simulink model "Multiphase_Buck"  (Simulink 6.1)
settings: Solver=ode23tb  SolverMode=SingleTasking  StartTime=0.0  StopTime=0.03  MaxStep=10e-6  RelTol=1e-3
libraries: powerlib x14
settings Model: Creator=patrice  LastModifiedBy=ThinkPad  ExtModeTrigMode=oneshot  ExtModeArmWhenConnect=off  ExtModeAutoUpdateStatusClock=off
settings DataIOCC: LimitDataPoints=off  SignalLoggingName=sigsOut
settings OptimizationCC: BooleanDataType=off
settings HardwareCC: TargetUnknown=on
settings RTWCC: TemplateMakefile=grt_unix.tmf

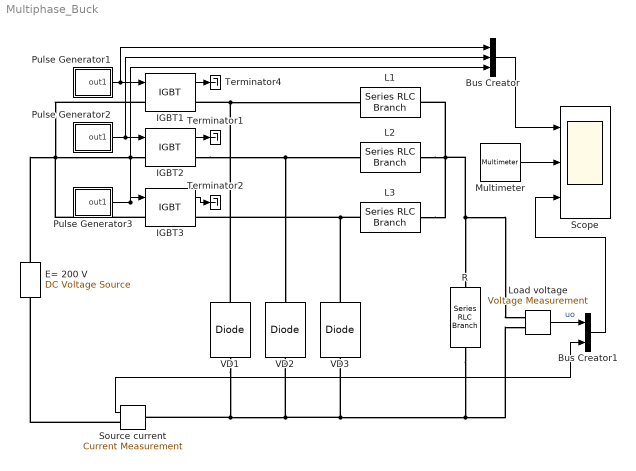
== system Multiphase_Buck ==
  Bus Creator : BusCreator  DialogController=Simulink.DDGSource_Bus  Inputs=3
  Bus Creator1 : BusCreator  DialogController=Simulink.DDGSource_Bus  Inputs=2
  E= 200 V : powerlib/Electrical Sources/DC Voltage Source  Description=source block  Orientation=up  Amplitude=200  Measurements=None
      settings: AttributesFormatString=\n
  IGBT1 : powerlib/Power Electronics/IGBT  Ron=0.5  Lon=1e-6  Vf=0  Tf=1e-6  Tt=1e-6  IC=0  Rs=10  Cs=1e-7  Measurements=on
      settings: AttributesFormatString=\n
  IGBT2 : powerlib/Power Electronics/IGBT  Ron=0.5  Lon=1e-6  Vf=0  Tf=1e-6  Tt=1e-6  IC=0  Rs=10  Cs=1e-7  Measurements=on
      settings: AttributesFormatString=\n
  IGBT3 : powerlib/Power Electronics/IGBT  Ron=0.5  Lon=1e-6  Vf=0  Tf=1e-6  Tt=1e-6  IC=0  Rs=10  Cs=1e-7  Measurements=on
      settings: AttributesFormatString=\n
  L1 : powerlib/Elements/Series RLC Branch  PhysicalDomain=powersysdomain  SubClassName=unknown  LeftPortType=p1  RightPortType=p1  LConnTagsString=__new0  RConnTagsString=__new0  Resistance=0  Inductance=5e-03  Capacitance=inf  Measurements=Branch current
  L2 : powerlib/Elements/Series RLC Branch  PhysicalDomain=powersysdomain  SubClassName=unknown  LeftPortType=p1  RightPortType=p1  LConnTagsString=__new0  RConnTagsString=__new0  Resistance=0  Inductance=5e-03  Capacitance=inf  Measurements=Branch current
  L3 : powerlib/Elements/Series RLC Branch  PhysicalDomain=powersysdomain  SubClassName=unknown  LeftPortType=p1  RightPortType=p1  LConnTagsString=__new0  RConnTagsString=__new0  Resistance=0  Inductance=5e-03  Capacitance=inf  Measurements=Branch current
  Load voltage : powerlib/Measurements/Voltage Measurement  Tag=PoWeRsYsTeMmEaSuReMeNt  PhasorSimulation=off  OutputType=Magnitude  PSBequivalent=0
  Multimeter : powerlib/Measurements/Multimeter  PhasorSimulation=off  OutputType=Complex  sel=[1 2 3]  L=3  Gain=[1 1 1]  yselected={'Ib: L1','Ib: L2','Ib: L3'};  PSBOutputType=1  PSBequivalent=0  AxesSetting=[0,0.1,-100,100]  Display=0  SavedBlockNames=-11
  Pulse Generator1 : Subsystem  mask(Pulse Generator){period=1e-3, duty=20, amplitude=1, start=0}
      mask prompts: period "Period (secs):"; duty "Duty cycle (% of period):"; start "Start time:"
      mask help: Pulse Generator
      mask Help: Pulse generator which ensures pulse transitions are hit. Provides a vector of pulses when the height is entered as a vector.  Unmask to see how it works.
      mask Display: plot(0,0,100,100,[95,90,90,75,75,60,60,45,45,30,30,15,15,5],[25,25,75,75,25,25,75,75,25,25,75,75,25,25]);
  Pulse Generator2 : Subsystem  mask(Pulse Generator){period=1e-3, duty=20, amplitude=1, start=3.3e-4}
      mask prompts: period "Period (secs):"; duty "Duty cycle (% of period):"; start "Start time:"
      mask help: Pulse Generator
      mask Help: Pulse generator which ensures pulse transitions are hit. Provides a vector of pulses when the height is entered as a vector.  Unmask to see how it works.
      mask Display: plot(0,0,100,100,[95,90,90,75,75,60,60,45,45,30,30,15,15,5],[25,25,75,75,25,25,75,75,25,25,75,75,25,25]);
  Pulse Generator3 : Subsystem  mask(Pulse Generator){period=1e-3, duty=20, amplitude=1, start=6.7e-4}
      mask prompts: period "Period (secs):"; duty "Duty cycle (% of period):"; start "Start time:"
      mask help: Pulse Generator
      mask Help: Pulse generator which ensures pulse transitions are hit. Provides a vector of pulses when the height is entered as a vector.  Unmask to see how it works.
      mask Display: plot(0,0,100,100,[95,90,90,75,75,60,60,45,45,30,30,15,15,5],[25,25,75,75,25,25,75,75,25,25,75,75,25,25]);
  R : powerlib/Elements/Series RLC Branch  Orientation=down  PhysicalDomain=powersysdomain  SubClassName=unknown  LeftPortType=p1  RightPortType=p1  LConnTagsString=__new0  RConnTagsString=__new0  Resistance=2  Inductance=0  Capacitance=inf  Measurements=None
  Scope : Scope  NumInputPorts=3
      settings: TimeRange=0.01  YMin=-1~-10~0  YMax=2~40~100  DataFormat=Array  MaxDataPoints=500000
  Source current : powerlib/Measurements/Current Measurement  Orientation=left  PhasorSimulation=off  OutputType=Complex  PSBequivalent=0
  Terminator1 : Terminator
  Terminator2 : Terminator
  Terminator4 : Terminator
  VD1 : powerlib/Power Electronics/Diode  Orientation=up  Ron=0.5  Lon=1e-9  Vf=0  IC=0  Rs=inf  Cs=0.1e-6  Measurements=off
  VD2 : powerlib/Power Electronics/Diode  Orientation=up  Ron=0.5  Lon=1e-9  Vf=0  IC=0  Rs=inf  Cs=0.1e-6  Measurements=off
  VD3 : powerlib/Power Electronics/Diode  Orientation=up  Ron=0.5  Lon=1e-9  Vf=0  IC=0  Rs=inf  Cs=0.1e-6  Measurements=off
  wires:
  Load voltage/1 -> Bus Creator1/1  "uo"
  Pulse Generator1/1(out1) -> IGBT1/1, Bus Creator/1
  IGBT1/1 -> Terminator4/1
  Pulse Generator2/1(out1) -> IGBT2/1, Bus Creator/2
  IGBT2/1 -> Terminator1/1
  IGBT3/1 -> Terminator2/1
  Bus Creator/1 -> Scope/1
  Multimeter/1 -> Scope/2
  Pulse Generator3/1(out1) -> IGBT3/1, Bus Creator/3
  Source current/1 -> Bus Creator1/2
  Bus Creator1/1 -> Scope/3
  connections:
  VD1/LConn1 -- VD2/LConn1 -- VD3/LConn1 -- R/RConn1 -- Load voltage/LConn2 -- Source current/LConn1
  IGBT1/LConn1 -- IGBT2/LConn1 -- IGBT3/LConn1 -- E= 200 V/RConn1
  VD1/RConn1 -- IGBT1/RConn1 -- L1/LConn1
  IGBT2/RConn1 -- VD2/RConn1 -- L2/LConn1
  L3/LConn1 -- IGBT3/RConn1 -- VD3/RConn1
  R/LConn1 -- Load voltage/LConn1 -- L1/RConn1 -- L2/RConn1 -- L3/RConn1
  Source current/RConn1 -- E= 200 V/LConn1

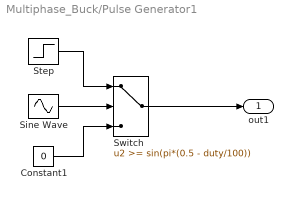
== system Multiphase_Buck/Pulse Generator1 ==
  Constant1 : Constant  Value=0
  Sine Wave : Sin  Frequency=2*pi./period  Phase=-2*pi*(start./period + duty/200 - 1/4)  SampleTime=0
  Step : Step  Time=start  After=amplitude  SampleTime=0
  Switch : Switch  Threshold=sin(pi*(0.5 - duty/100))  SaturateOnIntegerOverflow=on  InputSameDT=on
  out1 : Outport  InitialOutput=0
  wires:
  Step/1 -> Switch/1
  Constant1/1 -> Switch/3
  Switch/1 -> out1/1
  Sine Wave/1 -> Switch/2

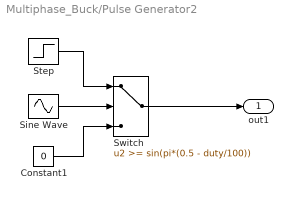
== system Multiphase_Buck/Pulse Generator2 ==
  Constant1 : Constant  Value=0
  Sine Wave : Sin  Frequency=2*pi./period  Phase=-2*pi*(start./period + duty/200 - 1/4)  SampleTime=0
  Step : Step  Time=start  After=amplitude  SampleTime=0
  Switch : Switch  Threshold=sin(pi*(0.5 - duty/100))  SaturateOnIntegerOverflow=on  InputSameDT=on
  out1 : Outport  InitialOutput=0
  wires:
  Step/1 -> Switch/1
  Constant1/1 -> Switch/3
  Switch/1 -> out1/1
  Sine Wave/1 -> Switch/2

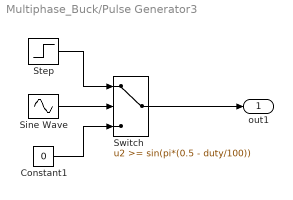
== system Multiphase_Buck/Pulse Generator3 ==
  Constant1 : Constant  Value=0
  Sine Wave : Sin  Frequency=2*pi./period  Phase=-2*pi*(start./period + duty/200 - 1/4)  SampleTime=0
  Step : Step  Time=start  After=amplitude  SampleTime=0
  Switch : Switch  Threshold=sin(pi*(0.5 - duty/100))  SaturateOnIntegerOverflow=on  InputSameDT=on
  out1 : Outport  InitialOutput=0
  wires:
  Step/1 -> Switch/1
  Constant1/1 -> Switch/3
  Switch/1 -> out1/1
  Sine Wave/1 -> Switch/2
